simulink library "Wall_with_Window"  (R2018b)
settings: Solver=ode45  StartTime=0.0  StopTime=10.0  RelTol=1e-3  EnableMultiTasking=on
libraries: carnot x2
settings Model: Creator=bernd.hafner  LastModifiedBy=drhf
settings DataIOCC: LimitDataPoints=on  SaveFormat=Array  SignalLoggingSaveFormat=ModelDataLogs
settings OptimizationCC: ExpressionDepthLimit=2147483647  LifeSpan=inf
settings DebuggingCC: UnderspecifiedInitializationDetection=Classic  MergeDetectMultiDrivingBlocksExec=none  SolverPrmCheckMsg=warning  FcnCallInpInsideContextMsg=warning  StateNameClashWarn=warning  SFUnexpectedBacktrackingDiag=warning  SFNoUnconditionalDefaultTransitionDiag=warning  SFExecutionAtInitializationDiag=none
settings HardwareCC: ProdBitPerPointer=32  ProdBitPerSizeT=32  ProdBitPerPtrDiffT=32  ProdLargestAtomicFloat=None  ProdIntDivRoundTo=Undefined  ProdEndianess=Unspecified  ProdWordSize=32  ProdHWDeviceType=32-bit Generic
settings ModelReferenceCC: PropagateSignalLabelsOutOfModel=off
settings SFSimCC: SimUseLocalCustomCode=off
settings RTWCC: RTWUseLocalCustomCode=off
settings CodeAppCC: StateflowObjectComments=on
settings GRTTargetCC: TargetLangStandard=C89/C90 (ANSI)  GeneratePreprocessorConditionals=Disable all  CombineOutputUpdateFcns=off  GRTInterface=on
settings ConfigComp: CovMetricSettings=dw  CovHtmlReporting=on  CovSaveCumulativeToWorkspaceVar=on  CovSaveSingleToWorkspaceVar=on  CovExternalEMLEnable=off

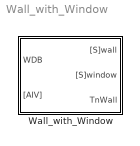
== system Wall_with_Window ==
  Wall_with_Window : Subsystem  mask(outer wall with window){wallsize=[2.5 5], windowsize=[1 2], frame=0.1, pos=0, t0=20, tau=1000*3600, g=0.7}
      mask prompts: wallsize "size of wall[m] [height width]"; windowsize "size of window[m] [height width]"; frame "part of frame of the window-surface (0..1)"; pos "azimut of wall (0=south, east= -90)]"; t0 "initial temperature [degree centigrade]"; tau "time-constant of wall and window [s]"; g "energy transmission of window"
      mask help:
      | This is the model of an outer wall with window.
      | first element of the vector = layer to surrounding
      | last element of the vector = layer to room
      mask init:
      | pos = [90 pos 0]; % position is [inclination azimut rotation]
      mask Help: web(fullfile(path_carnot('help'),'Wall_with_Window.html'),'-helpbrowser')

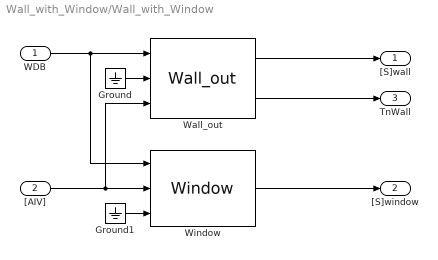
== system Wall_with_Window/Wall_with_Window ==
  WDB : Inport
  "[AIV]" : Inport  Port=2
  Ground : Ground
  Ground1 : Ground
  Wall_out : carnot/Basic/Thermal_Models/Wall_out  wallsize=[wallsize(1), wallsize(2)-windowsize(1)*windowsize(2)/wallsize(1)]  pos=pos  t0=t0  d=[0.1 0.38]  cond=[0.04 0.79]  cwall=[0.28 0.28]*3600  rho=[900 1800]  reflectground=0.3  abs_emiss=[0.65 0.97 0.96]  tau=tau  dactive=-1
      settings: SourceProductName=Carnot
  Window : carnot/Basic/Thermal_Models/Window  pos=pos  windowsize=windowsize  frame=frame  Ug=1.8  gvalue=g  tauzero=g*0.95  numpanes=2  d=[0.004 0.004]  rho=[2500 2500]  cp="[1008  1008]"  t0=t0  misc=[0.2 0.1 1 1]  shad_type=No shading  type_glazing=double glazing normal  tau_shad=0.01  bli_a=0.05  bli_b=1  bli_c=0.05  bli_d=0.05  bli_alpha=90  bli_refl=0.2
      settings: SourceProductName=Carnot
  "[S]wall" : Outport
  "[S]window" : Outport  Port=2
  TnWall : Outport  Port=3
  wires:
  Wall_out/2 -> TnWall/1
  WDB/1 -> Window/1, Wall_out/1
  "[AIV]"/1 -> Wall_out/3, Window/2
  Ground/1 -> Wall_out/2
  Wall_out/1 -> "[S]wall"/1
  Window/1 -> "[S]window"/1
  Ground1/1 -> Window/3
